simulink model "CorW_TestBed_org"  (Simulink 10.0)
settings: Solver=FixedStepDiscrete  StartTime=0.0  StopTime=1  FixedStep=1  RelTol=1e-3  EnableMultiTasking=on
undefined symbols (not defined in the file): MWS
libraries: Lib_Cntrl_CorrectedGasFlow_TMATS x1
settings Model: Creator=jwchapm2  LastModifiedBy=annonymous
settings DataIOCC: LimitDataPoints=on
settings OptimizationCC: ExpressionDepthLimit=2147483647
settings DebuggingCC: SolverPrmCheckMsg=warning  StateNameClashWarn=warning
settings GRTTargetCC: GeneratePreprocessorConditionals=Disable all  CombineOutputUpdateFcns=on  GRTInterface=off
settings ConfigComp: CovExternalEMLEnable=off

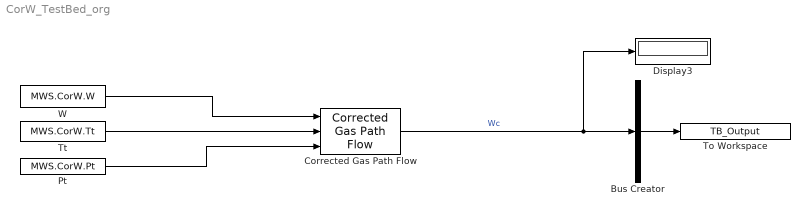
== system CorW_TestBed_org ==
  Bus Creator : BusCreator  Inputs=1
  Corrected Gas Path Flow : Lib_Cntrl_CorrectedGasFlow_TMATS/Corrected Gas Path Flow  C_TSTD_M=MWS.CorW.TST  C_PSTD_M=MWS.CorW.PST
  Display3 : Display
  Pt : Constant  Value=MWS.CorW.Pt
  To Workspace : ToWorkspace  VariableName=TB_Output  SampleTime=-1
  Tt : Constant  Value=MWS.CorW.Tt
  W : Constant  Value=MWS.CorW.W
  wires:
  W/1 -> Corrected Gas Path Flow/1
  Tt/1 -> Corrected Gas Path Flow/2
  Pt/1 -> Corrected Gas Path Flow/3
  Corrected Gas Path Flow/1 -> Display3/1, Bus Creator/1  "Wc"
  Bus Creator/1 -> To Workspace/1
